simulink model "poisson"  (R2023b)
settings: Solver=ode45  StartTime=0  StopTime=30  FixedStep=1  RelTol=1e-3
undefined symbols (not defined in the file): m, n
settings Model: Creator=anruk  LastModifiedBy=anruk

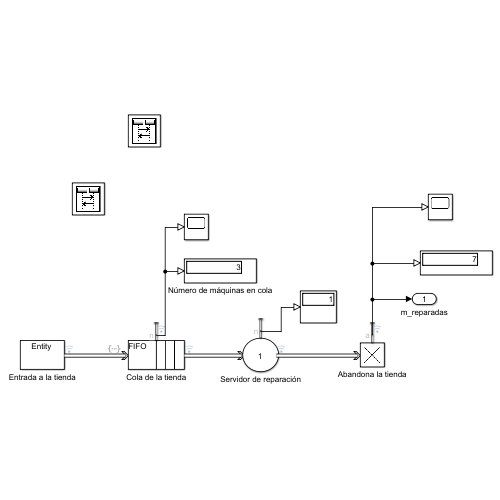
[thumbnail: Simulink's stored preview of the top-level diagram]
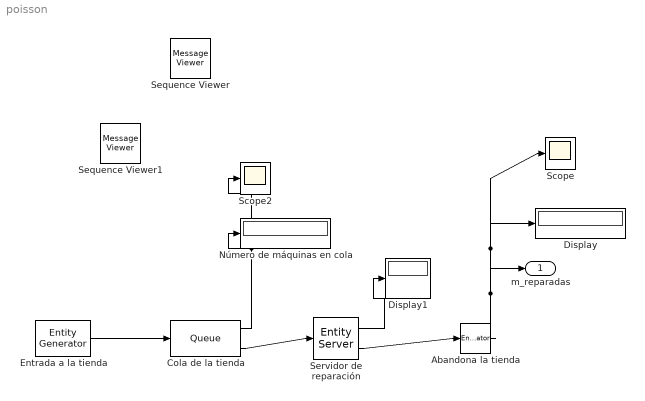
== system poisson ==
  Abandona la tienda : EntityTerminator  InputPortMessageModes=m  NumberEntitiesArrived=on
      settings: OutputPortMap=o0
  Cola de la tienda : Queue  InputPortMessageModes=m  OutputPortMessageModes=n,m  Capacity=10  EntryAction=entity.MaquinaTipo = randi([1,5]);  NumberEntitiesInBlock=on
      settings: OutputPortMap=o1,o5
  Display : Display
  Display1 : Display
  Entrada a la tienda : EntityGenerator  OutputPortMessageModes=m  TimeSource=MATLAB action  IntergenerationTimeAction=|  GenerateEntityAtSimulationStart=off  AttributeName=MaquinaTipo  EntityType=Structured  EntityTypeName=Entity
      | % Distribucion de poisson con media 2
      | dt = poissrnd(2);
  Número de máquinas en cola : Display
  Scope : Scope
  Scope2 : Scope
  Sequence Viewer : MessageViewer  History=1000  SavedRootId=#
  Sequence Viewer1 : MessageViewer  History=1000  SavedRootId=#
  Servidor de reparación : EntityServer  InputPortMessageModes=m  OutputPortMessageModes=n,m  Capacity=1  ServiceTimeSource=MATLAB action  ServiceTimeAction=|  NumberEntitiesInBlock=on
      | % Distribucion de poisson con media 1,2,3,4 o 5 
      | % Dependiendo del tipo de máquina
      | dt = poissrnd(entity.MaquinaTipo);
      settings: OutputPortMap=o1,o9
  m_reparadas : Outport
  wires:
  Entrada a la tienda/1 -> Cola de la tienda/1
  Cola de la tienda/2 -> Servidor de reparación/1
  Servidor de reparación/2 -> Abandona la tienda/1
  Abandona la tienda/1 -> Scope/1, Display/1, m_reparadas/1
  Cola de la tienda/1 -> Número de máquinas en cola/1, Scope2/1
  Servidor de reparación/1 -> Display1/1
